simulink model "Bio_Continuous"  (R2020b)
settings: Solver=daessc  StartTime=0.0  StopTime=100  RelTol=1e-3
settings Model: SimulationMode=accelerator  Creator=César-Garech  LastModifiedBy=César-Garech

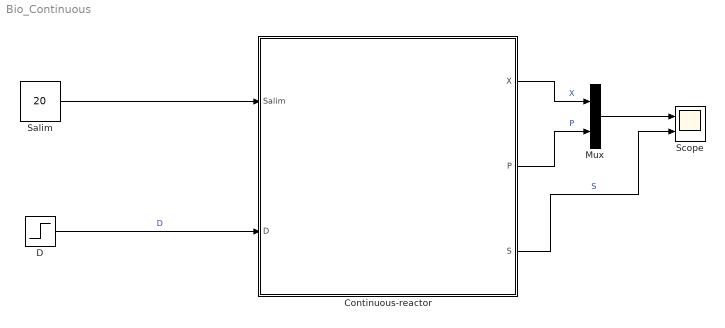
== system Bio_Continuous ==
  Continuous-reactor : Subsystem
      mask Display: image('biorreactor.png'); % Use "Edit Image" on toolstrip to change.
  D : Step  Time=5  After=0.15  SampleTime=0
  Mux : Mux  Inputs=2
  Salim : Constant  Value=20  VectorParams1D=off  SampleTime=-1
  Scope : Scope  NumInputPorts=2
  wires:
  Continuous-reactor/3(S) -> Scope/2  "S"
  Salim/1 -> Continuous-reactor/1(Salim)
  Continuous-reactor/2(P) -> Mux/2  "P"
  Continuous-reactor/1(X) -> Mux/1  "X"
  Mux/1 -> Scope/1
  D/1 -> Continuous-reactor/2(D)  "D"

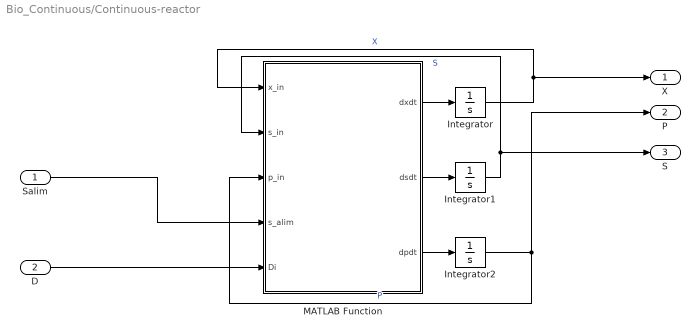
== system Bio_Continuous/Continuous-reactor ==
  Salim : Inport
  D : Inport  Port=2
  Integrator : Integrator  InitialCondition=0.01
  Integrator1 : Integrator  InitialCondition=20
  Integrator2 : Integrator
  MATLAB Function : MATLAB Function  TreatAsAtomicUnit=on
  X : Outport
  P : Outport  Port=2
  S : Outport  Port=3
  wires:
  MATLAB Function/3(dpdt) -> Integrator2/1
  Integrator/1 -> X/1, MATLAB Function/1(x_in)  "X"
  Integrator2/1 -> P/1, MATLAB Function/3(p_in)  "P"
  MATLAB Function/2(dsdt) -> Integrator1/1
  MATLAB Function/1(dxdt) -> Integrator/1
  Integrator1/1 -> MATLAB Function/2(s_in), S/1  "S"
  Salim/1 -> MATLAB Function/4(s_alim)
  D/1 -> MATLAB Function/5(Di)

== matlab function Bio_Continuous/Continuous-reactor/MATLAB Function ==
  data: x_in input; dxdt output; s_in input; p_in input; s_alim input; dsdt output; dpdt output; Di input
function [dxdt, dsdt,dpdt] =Bio_Continuous(x_in,s_in,p_in,s_alim,Di)

%Definir Parámetros
umax=0.75;%h^-1Velocidad de crecimiento máximo
Ks=0.08; %Afininidad por el sustrato
Smax=30; %Sustrato máximo que inhibie el crecimiento
Yxs=0.8;% (gX/gS) rendimiento de biomasa en sustrato
ms=0.00001; %constante de mantenimiento
alfa=0.05; %constante asociada al crecimiento
beta=0.002; %constante no asociada al crecimiento

%Condiciones iniciales
x=x_in;
s=s_in;
p=p_in;
D=Di;


%Ecuaciones constitutivas
u=umax*(s/(Ks+s)*(1-(s/Smax))); %h^-1
Rx=u*x;
Rs=(u/(Yxs)+ms)*x;
Rp=(alfa*u+beta)*x;

%Balances
dxdt=Rx-D*x;
dsdt=-Rs+D*(s_alim-s);
dpdt=Rp-D*p;


end
